simulink model "Sistema_Lineal_Equivalente"  (R2024b)
settings: Solver=VariableStepAuto  StartTime=0.0  StopTime=10.0  RelTol=1e-3
values from neighbouring files (symbols this model uses):
  alpha_cu = 3.9 *10^-3    (= 0.0039)    [parametros.m]
  b_eq = b_m + (1/r^2) * b_l    (= 2.19444444444e-05)    [parametros.m]
  C_ts = 0.818    [parametros.m]
  J_eq = J_m + (1/r^2) * J_l    (= 4.58263888889e-05)    [parametros.m]
  k_l = m * l_cm + m_l* l_l    (= 1)    [parametros.m]
  L_d = 6.6 * 10^-3    (= 0.0066)    [parametros.m]
  L_q = 5.8 * 10^-3    (= 0.0058)    [parametros.m]
  lambda_m = 0.016    [parametros.m]
  P_p = 3    [parametros.m]
  r = 120    [parametros.m]
  R_s_40 = 1.02    [parametros.m]
  R_ts_amb = 146.7    [parametros.m]
  Temp_s_ref = 20    [parametros.m]
settings Model: Creator=nsorr  LastModifiedBy=nsorr

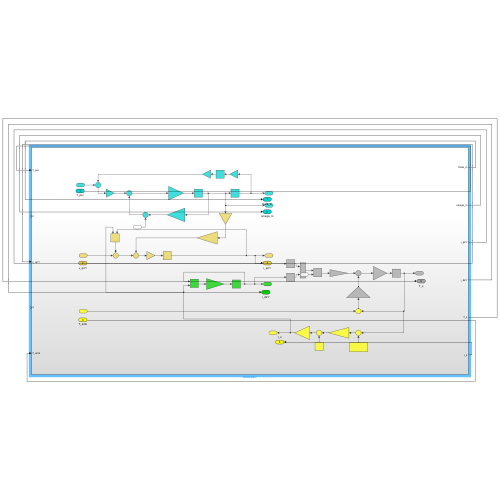
[thumbnail: Simulink's stored preview of the top-level diagram]
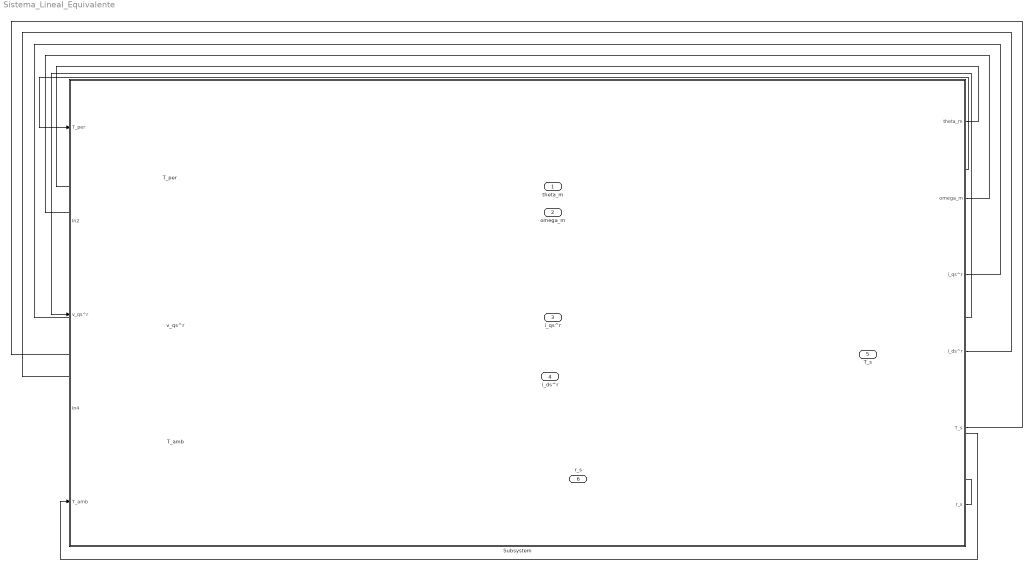
== system Sistema_Lineal_Equivalente ==
  T_per : Inport
  v_qs^r : Inport  Port=2
  T_amb : Inport  Port=3
  Subsystem : Subsystem
  theta_m : Outport
  omega_m : Outport  Port=2
  i_qs^r : Outport  Port=3
  i_ds^r : Outport  Port=4
  T_s : Outport  Port=5
  r_s : Outport  Port=6
  wires:
  T_per/1 -> Subsystem/1(T_per)
  v_qs^r/1 -> Subsystem/3(v_qs^r)
  T_amb/1 -> Subsystem/5(T_amb)
  Subsystem/1(theta_m) -> theta_m/1
  Subsystem/2(omega_m) -> omega_m/1
  Subsystem/3(i_qs^r) -> i_qs^r/1
  Subsystem/4(i_ds^r) -> i_ds^r/1
  Subsystem/5(T_s) -> T_s/1
  Subsystem/6(r_s) -> r_s/1

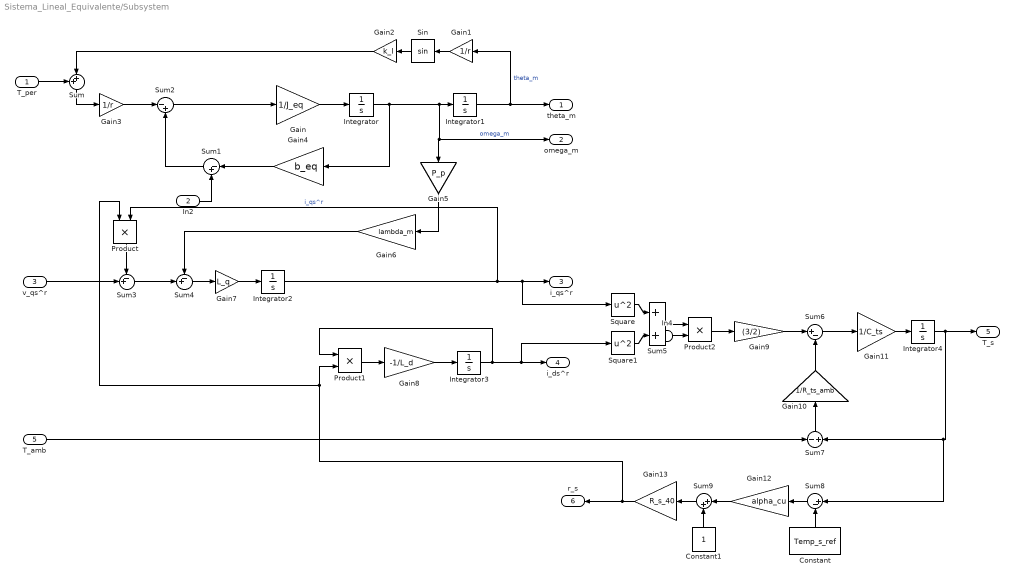
== system Sistema_Lineal_Equivalente/Subsystem ==
  T_per : Inport
  In2 : Inport  Port=2
  v_qs^r : Inport  Port=3
  In4 : Inport  Port=4
  T_amb : Inport  Port=5
  Constant : Constant  Value=Temp_s_ref
  Constant1 : Constant
  Gain : Gain  Gain=1/J_eq
  Gain1 : Gain  Gain=1/r
  Gain10 : Gain  Gain=1/R_ts_amb
  Gain11 : Gain  Gain=1/C_ts
  Gain12 : Gain  Gain=alpha_cu
  Gain13 : Gain  Gain=R_s_40
  Gain2 : Gain  Gain=k_l
  Gain3 : Gain  Gain=1/r
  Gain4 : Gain  Gain=b_eq
  Gain5 : Gain  Gain=P_p
  Gain6 : Gain  Gain=lambda_m
  Gain7 : Gain  Gain=L_q
  Gain8 : Gain  Gain=-1/L_d
  Gain9 : Gain  Gain=(3/2)
  Integrator{,1..3} (4 alike) : Integrator
  Integrator4 : Integrator  InitialCondition=40
  Product : Product
  Product1 : Product
  Product2 : Product
  Sin : Trigonometry
  Square : Math  Operator=square
  Square1 : Math  Operator=square
  Sum : Sum  Inputs=++|
  Sum1 : Sum  Inputs=|-+
  Sum2 : Sum  Inputs=|-+
  Sum3 : Sum  Inputs=-+|
  Sum4 : Sum  Inputs=-+|
  Sum5 : Sum
  Sum6 : Sum  Inputs=|+-
  Sum7 : Sum  Inputs=-|+
  Sum8 : Sum  Inputs=|+-
  Sum9 : Sum  Inputs=|++
  theta_m : Outport
  omega_m : Outport  Port=2
  i_qs^r : Outport  Port=3
  i_ds^r : Outport  Port=4
  T_s : Outport  Port=5
  r_s : Outport  Port=6
  wires:
  Gain/1 -> Integrator/1
  In2/1 -> Sum1/2
  v_qs^r/1 -> Sum3/2
  Integrator3/1 -> Product1/1, i_ds^r/1, Square1/1
  Sum9/1 -> Gain13/1
  Square1/1 -> Sum5/2
  Sum7/1 -> Gain10/1
  Sum4/1 -> Gain7/1
  Gain6/1 -> Sum4/1
  Gain11/1 -> Integrator4/1
  Gain1/1 -> Sin/1
  Integrator4/1 -> T_s/1, Sum8/1, Sum7/2
  Sum8/1 -> Gain12/1
  Gain13/1 -> r_s/1, Product/1, Product1/2
  Gain4/1 -> Sum1/1
  Constant/1 -> Sum8/2
  Sum2/1 -> Gain/1
  Sum1/1 -> Sum2/2
  Sin/1 -> Gain2/1
  Integrator1/1 -> theta_m/1, Gain1/1  "theta_m"
  Gain5/1 -> Gain6/1
  Gain8/1 -> Integrator3/1
  Integrator/1 -> Gain4/1, omega_m/1, Gain5/1, Integrator1/1  "omega_m"
  Sum5/1 -> Product2/1
  Product2/1 -> Gain9/1
  Sum/1 -> Gain3/1
  Gain7/1 -> Integrator2/1
  Sum6/1 -> Gain11/1
  Gain10/1 -> Sum6/2
  Square/1 -> Sum5/1
  Integrator2/1 -> i_qs^r/1, Square/1, Product/2  "i_qs^r"
  Gain9/1 -> Sum6/1
  Gain3/1 -> Sum2/1
  T_amb/1 -> Sum7/1
  Constant1/1 -> Sum9/2
  Gain12/1 -> Sum9/1
  T_per/1 -> Sum/1
  Gain2/1 -> Sum/2
  Product1/1 -> Gain8/1
  Product/1 -> Sum3/1
  Sum3/1 -> Sum4/2
  In4/1 -> Product2/2
